simulink model "verificationGG"  (R2023b)
settings: Solver=ode5  StartTime=0.0  StopTime=5000  FixedStep=0.01  RelTol=1e-10  AbsTol=1e-11
values from neighbouring files (symbols this model uses):
  A_0 = A_B_LVLH*A_LVLH_ECI_0    [SAD_CALLER.m]    (also in veriAxilsym.m = eye(3))
  correct_g = [5.7   7.4   0      0     0 ... (first row only)    [SAD_CALLER.m]    (also in veriAxilsym.m)
  correct_h = [  0  -25.9     0       0      0 ... (first row only)    [SAD_CALLER.m]    (also in veriAxilsym.m)
  g_nm = [-29404.8 -1450.9     0      0     0 ... (first row only)    [SAD_CALLER.m]    (also in veriAxilsym.m)
  h_nm = [  0  4652.5      0      0       0 ... (first row only)    [SAD_CALLER.m]    (also in veriAxilsym.m)
  I = I_a+diag([0,4*M_a*x_cm^2,4*M_a*x_cm^2])+I_c+diag([0,M_c*d_cc_cm^2,M_c*d_cc_cm^2])+I_p+diag([0,6*M_p*(d_cc+d_cc_cm)^2,6*M_p*(d_cc-d_cc_cm)^2])    [SAD_CALLER.m]    (also in veriAxilsym.m = diag(I))
  Inv_I = inv(I)    [SAD_CALLER.m]    (also in veriAxilsym.m = pinv(I))
  J2 = 1.082626925638815e-3    (= 0.00108262692564)    [SAD_CALLER.m]    (also in veriAxilsym.m)
  m_sc_body = [1;1;1]*10e-3*M_tot/sqrt(3)    [SAD_CALLER.m]    (also in veriAxilsym.m)
  mu_E = 3.986004418e5    (= 398600.4418)    [SAD_CALLER.m]    (also in veriAxilsym.m = 398600)
  omega_E = 2*pi/(24*60*60)    (= 7.27220521664e-05)    [SAD_CALLER.m]    (also in veriAxilsym.m)
  omega_sc_0 = [0,0,n]    [SAD_CALLER.m]    (also in veriAxilsym.m = [0; 0; 0])
  R_E_eqtr = 6378.1363    [SAD_CALLER.m]    (also in veriAxilsym.m)
  rr_Esc_0 = s(end,(1:3))'    [SAD_CALLER.m]    (also in veriAxilsym.m = [7070.6; 0; 0])
  smith_norm = zeros(4,5)    [SAD_CALLER.m]    (also in veriAxilsym.m)
  theta_G0 = mod(theta_G_Winter_solstice+omega_E*t_elapsed,2*pi)    [SAD_CALLER.m]    (also in veriAxilsym.m)
  vv_Esc_0 = s(end,(4:6))'    [SAD_CALLER.m]    (also in veriAxilsym.m = [0; 7.4338; 0])
undefined symbols (not defined in the file or in its folder): omega_0
libraries: matrix_library x4, simulink_extras x1
settings Model: Creator=WinUser  LastModifiedBy=a1pab

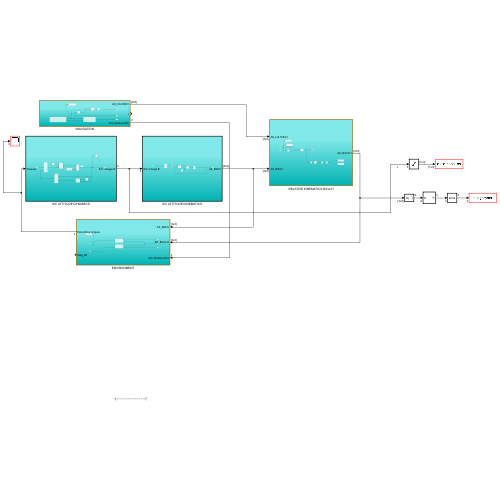
[thumbnail: Simulink's stored preview of the top-level diagram]
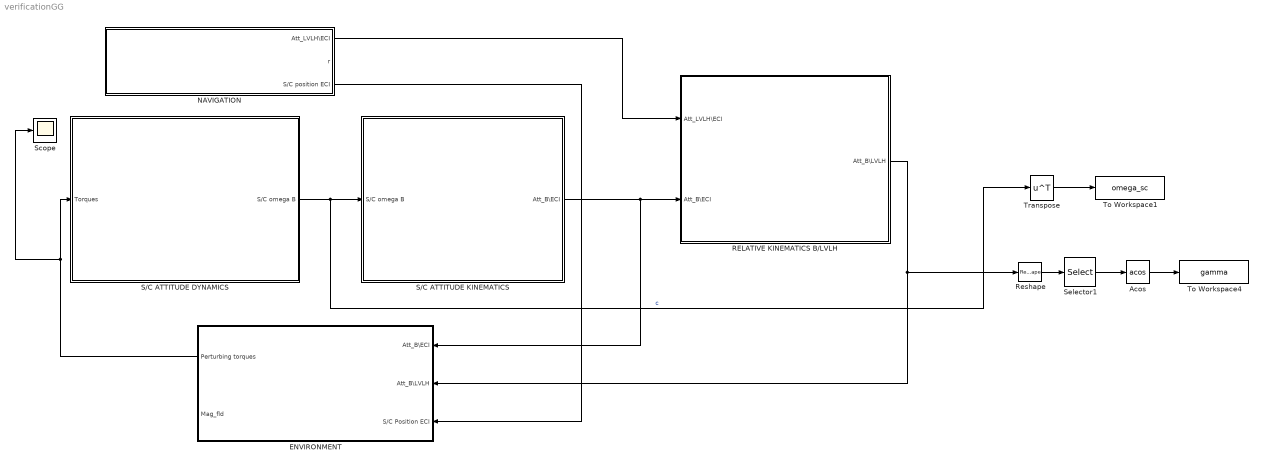
== system verificationGG ==
  Acos : Trigonometry  Operator=acos
  ENVIRONMENT : Subsystem
  NAVIGATION : Subsystem
  RELATIVE KINEMATICS B/LVLH : Subsystem
  Reshape : Reshape
  S/C ATTITUDE DYNAMICS : Subsystem
  S/C ATTITUDE KINEMATICS : Subsystem
  Scope : Scope
  Selector1 : Selector  InputPortWidth=9  IndexOptions=Index vector (dialog)  Indices=[1,5,9]  OutputSizes=1
  To Workspace1 : ToWorkspace  VariableName=omega_sc  SampleTime=-1
      settings: Save2DSignal=2-D array (concatenate along first dimension)
  To Workspace4 : ToWorkspace  VariableName=gamma  SampleTime=-1
      settings: Save2DSignal=2-D array (concatenate along first dimension)
  Transpose : Math  Operator=transpose
  wires:
  ? -> ?
  NAVIGATION/1(Att_LVLH\ECI) -> RELATIVE KINEMATICS B/LVLH/1(Att_LVLH\ECI)
  NAVIGATION/3(S/C position ECI) -> ENVIRONMENT/3(S/C Position ECI)
  RELATIVE KINEMATICS B/LVLH/1(Att_B\LVLH) -> Reshape/1, ENVIRONMENT/2(Att_B\LVLH)
  S/C ATTITUDE DYNAMICS/1(S/C omega B) -> Transpose/1, S/C ATTITUDE KINEMATICS/1(S/C omega B)  "c"
  Transpose/1 -> To Workspace1/1
  Selector1/1 -> Acos/1
  Reshape/1 -> Selector1/1
  Acos/1 -> To Workspace4/1
  S/C ATTITUDE KINEMATICS/1(Att_B\ECI) -> ENVIRONMENT/1(Att_B\ECI), RELATIVE KINEMATICS B/LVLH/2(Att_B\ECI)
  ENVIRONMENT/1(Perturbing torques) -> S/C ATTITUDE DYNAMICS/1(Torques), Scope/1

== system verificationGG/ENVIRONMENT ==
  Att_B\ECI : Inport
  Att_B\LVLH : Inport  Port=2
  S/C Position ECI : Inport  Port=3
  Gravity Gradient : Subsystem
  Magnetic Torque : Subsystem
  Sum : Sum  Inputs=+|+
  To Workspace1 : ToWorkspace  VariableName=ext_perturbations  SampleTime=-1
  Perturbing torques : Outport
  Mag_fld : Outport  Port=2
  wires:
  S/C Position ECI/1 -> Gravity Gradient/2(S/C Position), Magnetic Torque/1("[km]")
  Att_B\ECI/1 -> Magnetic Torque/2(True Attitude B\N)
  Att_B\LVLH/1 -> Gravity Gradient/1(Att_B\L)
  Gravity Gradient/1(GG_Torque) -> Sum/1
  Sum/1 -> To Workspace1/1, Perturbing torques/1
  Magnetic Torque/2(Mag_fld) -> Mag_fld/1

== system verificationGG/NAVIGATION ==
  LVLH Kinematics : Subsystem
  Matrix Multiply : Product  Multiplication=Matrix(*)
  S/C Orbit propagation : Subsystem
  Sqrt : Sqrt
  To Workspace4 : ToWorkspace  VariableName=position  SampleTime=-1
      settings: Save2DSignal=2-D array (concatenate along first dimension)
  Transpose : Math  Operator=transpose
  Att_LVLH\ECI : Outport
  r : Outport  Port=2
  S/C position ECI : Outport  Port=3
  wires:
  S/C Orbit propagation/2(S/C Velocity ECI) -> LVLH Kinematics/2(velocity)  "[km/s]"
  LVLH Kinematics/1(Att_LVLH\ECI) -> Att_LVLH\ECI/1
  Matrix Multiply/1 -> Sqrt/1
  Sqrt/1 -> r/1
  Transpose/1 -> Matrix Multiply/1
  S/C Orbit propagation/1(S/C Posiion ECI) -> To Workspace4/1, Matrix Multiply/2, Transpose/1, S/C position ECI/1, LVLH Kinematics/1(position)

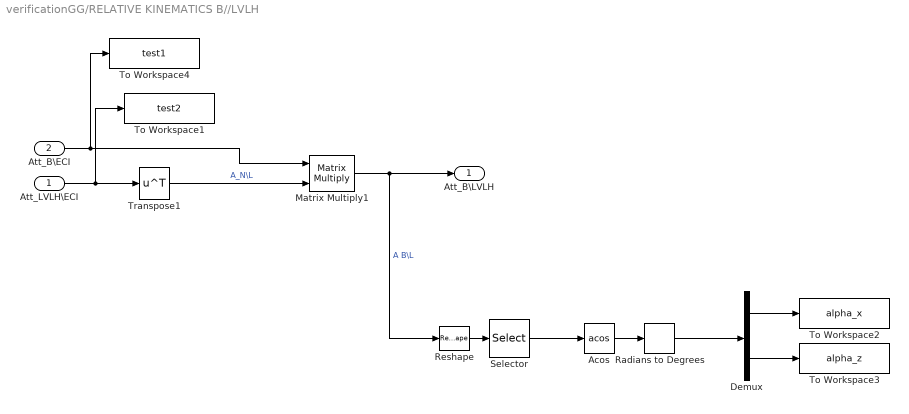
== system verificationGG/RELATIVE KINEMATICS B//LVLH ==
  Att_LVLH\ECI : Inport
  Att_B\ECI : Inport  Port=2
  Acos : Trigonometry  Operator=acos
  Demux : Demux  Outputs=2
  Matrix Multiply1 : Product  Multiplication=Matrix(*)
  Radians to Degrees : simulink_extras/Transformations/Radians to Degrees
  Reshape : Reshape
  Selector : Selector  InputPortWidth=9  IndexOptions=Index vector (dialog)  Indices=[1,9]  OutputSizes=1
  To Workspace1 : ToWorkspace  VariableName=test2  SampleTime=-1
      settings: Save2DSignal=2-D array (concatenate along first dimension)
  To Workspace2 : ToWorkspace  VariableName=alpha_x  SampleTime=-1
      settings: Save2DSignal=2-D array (concatenate along first dimension)
  To Workspace3 : ToWorkspace  VariableName=alpha_z  SampleTime=-1
      settings: Save2DSignal=2-D array (concatenate along first dimension)
  To Workspace4 : ToWorkspace  VariableName=test1  SampleTime=-1
      settings: Save2DSignal=2-D array (concatenate along first dimension)
  Transpose1 : Math  Operator=transpose
  Att_B\LVLH : Outport
  wires:
  Transpose1/1 -> Matrix Multiply1/2  "A_N\\L"
  Matrix Multiply1/1 -> Reshape/1, Att_B\LVLH/1  "A B\\L"
  Att_B\ECI/1 -> To Workspace4/1, Matrix Multiply1/1
  Att_LVLH\ECI/1 -> To Workspace1/1, Transpose1/1
  Demux/2 -> To Workspace3/1
  Demux/1 -> To Workspace2/1
  Selector/1 -> Acos/1
  Reshape/1 -> Selector/1
  Radians to Degrees/1 -> Demux/1
  Acos/1 -> Radians to Degrees/1

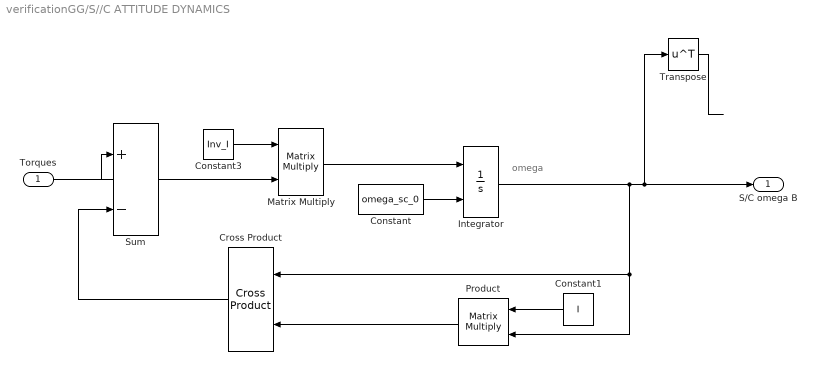
== system verificationGG/S//C ATTITUDE DYNAMICS ==
  note: omega
  Torques : Inport
  Constant : Constant  Value=omega_sc_0
  Constant1 : Constant  Value=I  VectorParams1D=off
  Constant3 : Constant  Value=Inv_I  VectorParams1D=off
  Cross Product : matrix_library/Cross Product
  Integrator : Integrator  InitialConditionSource=external  InitialCondition=omega_0
  Matrix Multiply : Product  Multiplication=Matrix(*)
  Product : Product  Multiplication=Matrix(*)
  Sum : Sum  Inputs=|+-
  Transpose : Math  Operator=transpose
  S/C omega B : Outport
  wires:
  Constant3/1 -> Matrix Multiply/1
  Constant/1 -> Integrator/2
  Sum/1 -> Matrix Multiply/2
  Cross Product/1 -> Sum/2
  Integrator/1 -> S/C omega B/1, Transpose/1, Cross Product/1, Product/2
  Constant1/1 -> Product/1
  Matrix Multiply/1 -> Integrator/1
  Torques/1 -> Sum/1
  Product/1 -> Cross Product/2
  Transpose/1 -> ?

== system verificationGG/S//C ATTITUDE KINEMATICS ==
  S/C omega B : Inport
  1st order orthon. : Subsystem
  Angular velocity tensor : Subsystem
  Constant3 : Constant  Value=A_0
  Gain : Gain  Gain=-1
  Integrator1 : Integrator  InitialConditionSource=external  InitialCondition=omega_0
  Matrix Multiply : Product  Multiplication=Matrix(*)
  Att_B\ECI : Outport
  wires:
  Constant3/1 -> Integrator1/2
  S/C omega B/1 -> Angular velocity tensor/1(In1)  "omega B\\N"
  1st order orthon./1(Out1) -> Att_B\ECI/1, Matrix Multiply/2  "True Attitude B\\N"
  Integrator1/1 -> 1st order orthon./1(In1)
  Matrix Multiply/1 -> Integrator1/1
  Gain/1 -> Matrix Multiply/1
  Angular velocity tensor/1(Out1) -> Gain/1

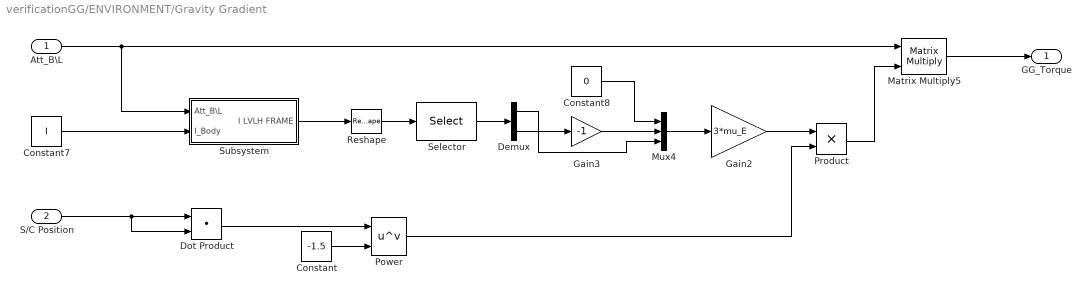
== system verificationGG/ENVIRONMENT/Gravity Gradient ==
  Att_B\L : Inport
  S/C Position : Inport  Port=2
  Constant : Constant  Value=-1.5
  Constant7 : Constant  Value=I
  Constant8 : Constant  Value=0
  Demux : Demux  Outputs=2
  Dot Product : DotProduct  OutDataTypeStr=Inherit: Inherit via internal rule
  Gain2 : Gain  Gain=3*mu_E
  Gain3 : Gain  Gain=-1
  Matrix Multiply5 : Product  Multiplication=Matrix(*)
  Mux4 : Mux  Inputs=3
  Power : Math  Operator=pow
  Product : Product
  Reshape : Reshape
  Selector : Selector  InputPortWidth=9  IndexOptions=Index vector (dialog)  Indices=[2,3]  OutputSizes=1
  Subsystem : Subsystem
  GG_Torque : Outport
  wires:
  Selector/1 -> Demux/1
  Reshape/1 -> Selector/1
  Att_B\L/1 -> Subsystem/1(Att_B\L), Matrix Multiply5/1
  Mux4/1 -> Gain2/1
  Constant8/1 -> Mux4/1
  Demux/1 -> Mux4/3
  Matrix Multiply5/1 -> GG_Torque/1
  Demux/2 -> Gain3/1
  Gain3/1 -> Mux4/2
  Constant7/1 -> Subsystem/2(I_Body)
  Subsystem/1(I LVLH FRAME) -> Reshape/1
  Gain2/1 -> Product/1
  Product/1 -> Matrix Multiply5/2
  S/C Position/1 -> Dot Product/1, Dot Product/2
  Dot Product/1 -> Power/1
  Constant/1 -> Power/2
  Power/1 -> Product/2

== system verificationGG/ENVIRONMENT/Magnetic Torque ==
  "[km]" : Inport
  True Attitude B\N : Inport  Port=2
  Cartesian 2 spherical : Subsystem
  Constant1 : Constant  Value=m_sc_body
  MAGNETIC TORQUE in BODY : Subsystem
  MF_Torque : Outport
  Mag_fld : Outport  Port=2
  wires:
  "[km]"/1 -> Cartesian 2 spherical/1("[km]")
  Cartesian 2 spherical/1(LST) -> MAGNETIC TORQUE in BODY/1(local siderial time)
  Cartesian 2 spherical/2(Long) -> MAGNETIC TORQUE in BODY/2(longitude)  "[rad]"
  Cartesian 2 spherical/3(radius) -> MAGNETIC TORQUE in BODY/3(r)
  Constant1/1 -> MAGNETIC TORQUE in BODY/6(a)
  MAGNETIC TORQUE in BODY/1(M) -> MF_Torque/1
  Cartesian 2 spherical/4(lat) -> MAGNETIC TORQUE in BODY/4(latitude)  "[rad]"
  True Attitude B\N/1 -> MAGNETIC TORQUE in BODY/5(True_Att_B\N)
  MAGNETIC TORQUE in BODY/2(Mag_fld) -> Mag_fld/1

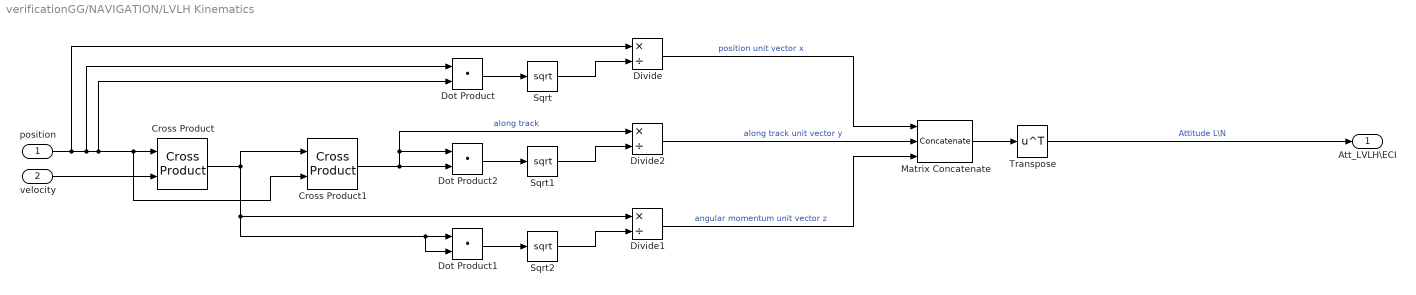
== system verificationGG/NAVIGATION/LVLH Kinematics ==
  position : Inport
  velocity : Inport  Port=2
  Cross Product : matrix_library/Cross Product
  Cross Product1 : matrix_library/Cross Product
  Divide : Product  Inputs=*/
  Divide1 : Product  Inputs=*/
  Divide2 : Product  Inputs=*/
  Dot Product : DotProduct  OutDataTypeStr=Inherit: Inherit via internal rule
  Dot Product1 : DotProduct  OutDataTypeStr=Inherit: Inherit via internal rule
  Dot Product2 : DotProduct  OutDataTypeStr=Inherit: Inherit via internal rule
  Matrix Concatenate : Concatenate  NumInputs=3  Mode=Multidimensional array  ConcatenateDimension=2
  Sqrt : Sqrt
  Sqrt1 : Sqrt
  Sqrt2 : Sqrt
  Transpose : Math  Operator=transpose
  Att_LVLH\ECI : Outport
  wires:
  Divide2/1 -> Matrix Concatenate/2  "along track unit vector y"
  Sqrt/1 -> Divide/2
  Cross Product/1 -> Dot Product1/2, Dot Product1/1, Divide1/1, Cross Product1/1
  Cross Product1/1 -> Divide2/1, Dot Product2/1, Dot Product2/2  "along track"
  Divide/1 -> Matrix Concatenate/1  "position unit vector x"
  position/1 -> Divide/1, Dot Product/1, Dot Product/2, Cross Product1/2, Cross Product/1
  velocity/1 -> Cross Product/2
  Sqrt2/1 -> Divide1/2
  Matrix Concatenate/1 -> Transpose/1
  Sqrt1/1 -> Divide2/2
  Divide1/1 -> Matrix Concatenate/3  "angular momentum unit vector z"
  Dot Product1/1 -> Sqrt2/1
  Dot Product/1 -> Sqrt/1
  Dot Product2/1 -> Sqrt1/1
  Transpose/1 -> Att_LVLH\ECI/1  "Attitude L\\N"

== system verificationGG/NAVIGATION/S//C Orbit propagation ==
  Constant5 : Constant  Value=vv_Esc_0
  Constant6 : Constant  Value=rr_Esc_0
  Integrator2 : Integrator  InitialConditionSource=external
  Integrator3 : Integrator  InitialConditionSource=external
  J2 perturbation : Subsystem
  Keplerian motion : Subsystem
  Sum : Sum  Inputs=|+-
  To Workspace : ToWorkspace  VariableName=RR_Esc  SampleTime=-1
  To Workspace1 : ToWorkspace  VariableName=VV_Esc  SampleTime=-1
  S/C Posiion ECI : Outport
  S/C Velocity ECI : Outport  Port=2
  wires:
  J2 perturbation/1(J2 acceleration) -> Sum/1
  Keplerian motion/1(Keplerian acceleration) -> Sum/2
  Constant5/1 -> Integrator2/2
  Integrator2/1 -> To Workspace1/1, S/C Velocity ECI/1, Integrator3/1  "dr"
  Constant6/1 -> Integrator3/2
  Sum/1 -> Integrator2/1  "ddr"
  Integrator3/1 -> S/C Posiion ECI/1, J2 perturbation/1(Position vector), Keplerian motion/1(Position vector), To Workspace/1  "r"

== system verificationGG/S//C ATTITUDE KINEMATICS/1st order orthon. ==
  In1 : Inport
  Gain1 : Gain  Gain=3/2
  Gain2 : Gain  Gain=1/2
  Matrix Multiply1 : Product  Multiplication=Matrix(*)
  Matrix Multiply2 : Product  Multiplication=Matrix(*)
  Sum1 : Sum  Inputs=|+-
  Transpose : Math  Operator=transpose
  Out1 : Outport
  wires:
  Gain1/1 -> Sum1/1
  In1/1 -> Matrix Multiply2/2, Transpose/1, Gain2/1, Gain1/1
  Transpose/1 -> Matrix Multiply1/2
  Matrix Multiply2/1 -> Sum1/2
  Matrix Multiply1/1 -> Matrix Multiply2/1
  Sum1/1 -> Out1/1
  Gain2/1 -> Matrix Multiply1/1

== system verificationGG/S//C ATTITUDE KINEMATICS/Angular velocity tensor ==
  In1 : Inport
  Constant : Constant  Value=0
  Demux1 : Demux  Outputs=3
  Gain3 : Gain  Gain=-1
  Gain4 : Gain  Gain=-1
  Gain5 : Gain  Gain=-1
  Mux3 : Mux  Inputs=3
  Mux4 : Mux  Inputs=3
  Mux5 : Mux  Inputs=3
  Vector Concatenate : Concatenate  NumInputs=3  Mode=Multidimensional array  ConcatenateDimension=2
  Out1 : Outport
  wires:
  In1/1 -> Demux1/1
  Constant/1 -> Mux3/1, Mux4/2, Mux5/3
  Demux1/3 -> Gain4/1, Mux3/2
  Demux1/2 -> Gain3/1, Mux5/1
  Gain3/1 -> Mux3/3
  Gain4/1 -> Mux4/1
  Mux4/1 -> Vector Concatenate/2
  Demux1/1 -> Gain5/1, Mux4/3
  Gain5/1 -> Mux5/2
  Mux5/1 -> Vector Concatenate/3
  Mux3/1 -> Vector Concatenate/1
  Vector Concatenate/1 -> Out1/1

== system verificationGG/ENVIRONMENT/Gravity Gradient/Subsystem ==
  Att_B\L : Inport
  I_Body : Inport  Port=2
  Matrix Multiply3 : Product  Multiplication=Matrix(*)
  Matrix Multiply4 : Product  Multiplication=Matrix(*)
  Transpose2 : Math  Operator=transpose
  I LVLH FRAME : Outport
  wires:
  Matrix Multiply3/1 -> I LVLH FRAME/1  "I LVLH FRAME"
  Matrix Multiply4/1 -> Matrix Multiply3/1
  I_Body/1 -> Matrix Multiply4/2
  Att_B\L/1 -> Transpose2/1, Matrix Multiply3/2
  Transpose2/1 -> Matrix Multiply4/1

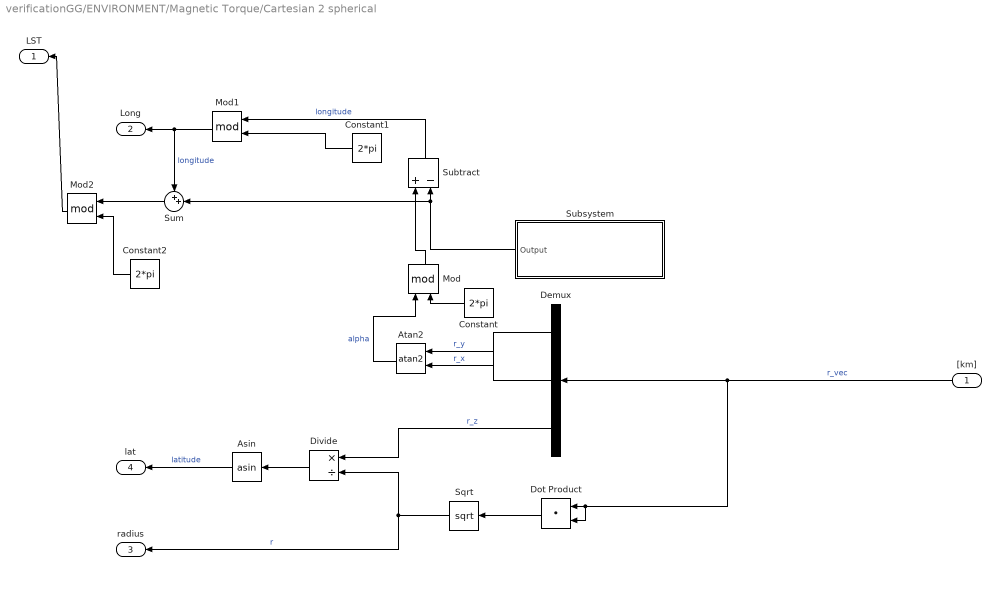
== system verificationGG/ENVIRONMENT/Magnetic Torque/Cartesian 2 spherical ==
  "[km]" : Inport
  Asin : Trigonometry  Operator=asin
  Atan2 : Trigonometry  Operator=atan2
  Constant : Constant  Value=2*pi
  Constant1 : Constant  Value=2*pi
  Constant2 : Constant  Value=2*pi
  Demux : Demux  Outputs=3
  Divide : Product  Inputs=*/
  Dot Product : DotProduct  OutDataTypeStr=Inherit: Inherit via internal rule
  Mod : Math  Operator=mod
  Mod1 : Math  Operator=mod
  Mod2 : Math  Operator=mod
  Sqrt : Sqrt
  Subsystem : Subsystem
  Subtract : Sum  Inputs=+-
  Sum : Sum  Inputs=++|
  LST : Outport
  Long : Outport  Port=2
  radius : Outport  Port=3
  lat : Outport  Port=4
  wires:
  "[km]"/1 -> Dot Product/2, Dot Product/1, Demux/1  "r_vec"
  Demux/2 -> Atan2/1  "r_y"
  Demux/1 -> Atan2/2  "r_x"
  Subsystem/1(Output) -> Sum/2, Subtract/2
  Dot Product/1 -> Sqrt/1
  Demux/3 -> Divide/1  "r_z"
  Sqrt/1 -> radius/1, Divide/2  "r"
  Divide/1 -> Asin/1
  Asin/1 -> lat/1  "latitude"
  Constant1/1 -> Mod1/2
  Subtract/1 -> Mod1/1  "longitude"
  Mod/1 -> Subtract/1
  Atan2/1 -> Mod/1  "alpha"
  Constant/1 -> Mod/2
  Mod1/1 -> Long/1, Sum/1  "longitude"
  Sum/1 -> Mod2/1
  Constant2/1 -> Mod2/2
  Mod2/1 -> LST/1

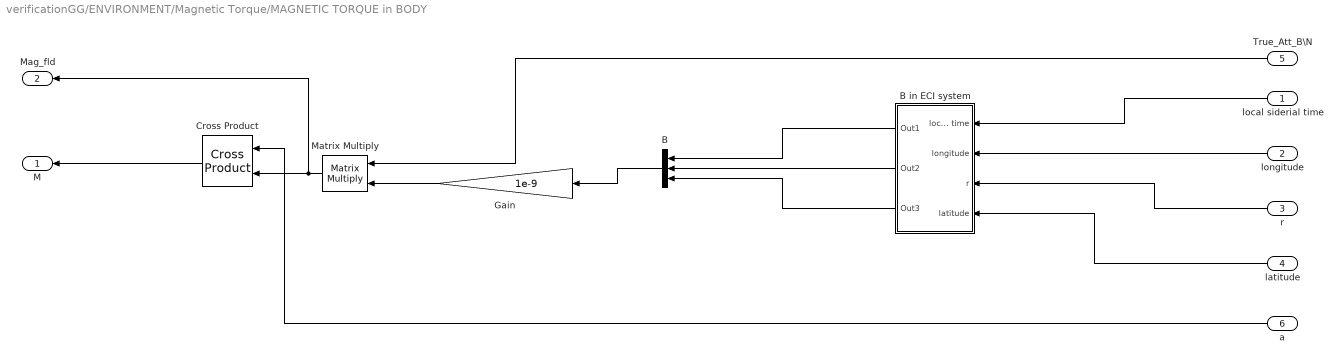
== system verificationGG/ENVIRONMENT/Magnetic Torque/MAGNETIC TORQUE in BODY ==
  local siderial time : Inport
  longitude : Inport  Port=2
  r : Inport  Port=3
  latitude : Inport  Port=4
  True_Att_B\N : Inport  Port=5
  a : Inport  Port=6
  B : Concatenate  NumInputs=3
  B in ECI system : Subsystem
  Cross Product : matrix_library/Cross Product
  Gain : Gain  Gain=1e-9
  Matrix Multiply : Product  Multiplication=Matrix(*)
  M : Outport
  Mag_fld : Outport  Port=2
  wires:
  B in ECI system/1(Out1) -> B/1
  a/1 -> Cross Product/1
  B in ECI system/2(Out2) -> B/2
  r/1 -> B in ECI system/3(r)
  local siderial time/1 -> B in ECI system/1(local siderial time)
  latitude/1 -> B in ECI system/4(latitude)
  B in ECI system/3(Out3) -> B/3
  Cross Product/1 -> M/1
  longitude/1 -> B in ECI system/2(longitude)
  B/1 -> Gain/1
  True_Att_B\N/1 -> Matrix Multiply/1
  Gain/1 -> Matrix Multiply/2
  Matrix Multiply/1 -> Mag_fld/1, Cross Product/2

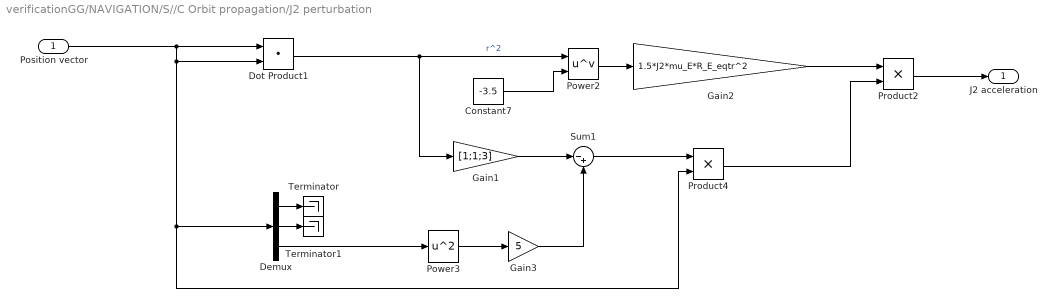
== system verificationGG/NAVIGATION/S//C Orbit propagation/J2 perturbation ==
  Position vector : Inport
  Constant7 : Constant  Value=-3.5
  Demux : Demux  Outputs=3
  Dot Product1 : DotProduct  OutDataTypeStr=Inherit: Inherit via internal rule
  Gain1 : Gain  Gain=[1;1;3]
  Gain2 : Gain  Gain=1.5*J2*mu_E*R_E_eqtr^2
  Gain3 : Gain  Gain=5
  Power2 : Math  Operator=pow
  Power3 : Math  Operator=square
  Product2 : Product
  Product4 : Product
  Sum1 : Sum  Inputs=|-+
  Terminator : Terminator
  Terminator1 : Terminator
  J2 acceleration : Outport
  wires:
  Gain3/1 -> Sum1/2
  Power2/1 -> Gain2/1
  Dot Product1/1 -> Power2/1, Gain1/1  "r^2"
  Demux/1 -> Terminator/1
  Gain1/1 -> Sum1/1
  Gain2/1 -> Product2/1
  Demux/3 -> Power3/1
  Power3/1 -> Gain3/1
  Product4/1 -> Product2/2
  Demux/2 -> Terminator1/1
  Constant7/1 -> Power2/2
  Product2/1 -> J2 acceleration/1
  Position vector/1 -> Demux/1, Product4/2, Dot Product1/2, Dot Product1/1
  Sum1/1 -> Product4/1

== system verificationGG/NAVIGATION/S//C Orbit propagation/Keplerian motion ==
  Position vector : Inport
  Constant : Constant  Value=-1.5
  Dot Product2 : DotProduct  OutDataTypeStr=Inherit: Inherit via internal rule
  Gain1 : Gain  Gain=mu_E
  Power : Math  Operator=pow
  Product1 : Product
  Keplerian acceleration : Outport
  wires:
  Position vector/1 -> Product1/2, Dot Product2/2, Dot Product2/1
  Power/1 -> Gain1/1
  Gain1/1 -> Product1/1
  Product1/1 -> Keplerian acceleration/1
  Constant/1 -> Power/2
  Dot Product2/1 -> Power/1  "r^2"

== system verificationGG/ENVIRONMENT/Magnetic Torque/Cartesian 2 spherical/Subsystem ==
  Clock : Clock
  Constant : Constant  Value=theta_G0
  Constant1 : Constant  Value=omega_E
  Constant2 : Constant  Value=2*pi
  Mod : Math  Operator=mod
  Product : Product
  Sum : Sum  Inputs=|++
  Output : Outport
  wires:
  Constant/1 -> Sum/1
  Product/1 -> Sum/2
  Clock/1 -> Product/2
  Sum/1 -> Mod/1  "theta_G(t)"
  Constant1/1 -> Product/1
  Constant2/1 -> Mod/2
  Mod/1 -> Output/1

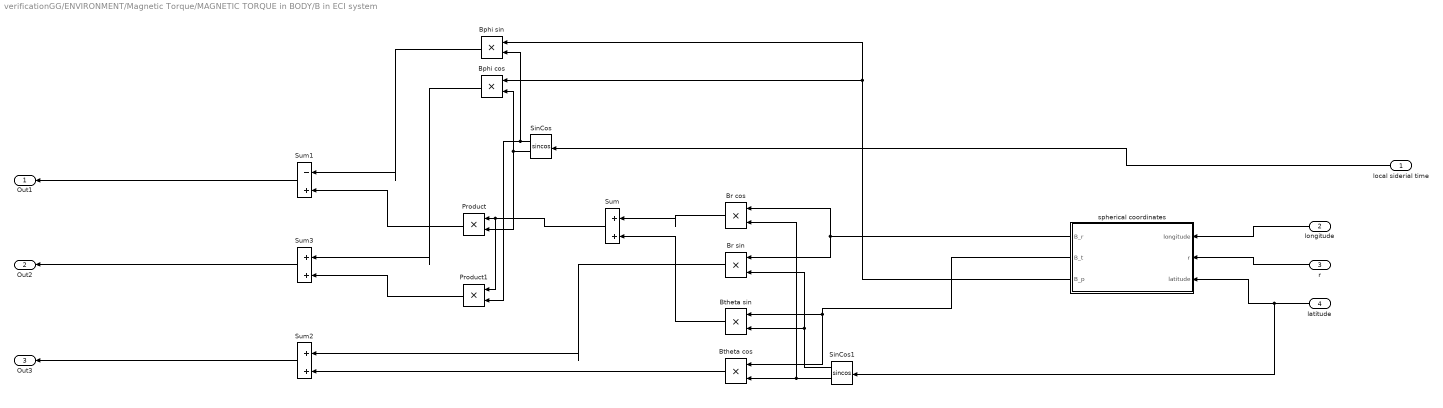
== system verificationGG/ENVIRONMENT/Magnetic Torque/MAGNETIC TORQUE in BODY/B in ECI system ==
  local siderial time : Inport
  longitude : Inport  Port=2
  r : Inport  Port=3
  latitude : Inport  Port=4
  Bphi cos : Product
  Bphi sin : Product
  Br cos : Product
  Br sin : Product
  Btheta cos : Product
  Btheta sin : Product
  Product : Product
  Product1 : Product
  SinCos : Trigonometry  Operator=sincos
  SinCos1 : Trigonometry  Operator=sincos
  Sum : Sum  Inputs=|++
  Sum1 : Sum  Inputs=|-+
  Sum2 : Sum  Inputs=|++
  Sum3 : Sum  Inputs=|++
  spherical coordinates : Subsystem
  Out1 : Outport
  Out2 : Outport  Port=2
  Out3 : Outport  Port=3
  wires:
  Sum3/1 -> Out2/1
  Sum1/1 -> Out1/1
  Bphi sin/1 -> Sum1/1
  Btheta sin/1 -> Sum/2
  Sum2/1 -> Out3/1
  Product1/1 -> Sum3/2
  SinCos1/2 -> Btheta cos/2, Br cos/2
  r/1 -> spherical coordinates/2(r)
  latitude/1 -> SinCos1/1, spherical coordinates/3(latitude)
  spherical coordinates/1(B_r) -> Br cos/1, Br sin/1
  Br sin/1 -> Sum2/1
  longitude/1 -> spherical coordinates/1(longitude)
  local siderial time/1 -> SinCos/1
  spherical coordinates/2(B_t) -> Btheta sin/1, Btheta cos/1
  Sum/1 -> Product1/1, Product/1
  Br cos/1 -> Sum/1
  Btheta cos/1 -> Sum2/2
  SinCos1/1 -> Btheta sin/2, Br sin/2
  SinCos/2 -> Bphi cos/2, Product/2
  Bphi cos/1 -> Sum3/1
  SinCos/1 -> Bphi sin/2, Product1/2
  Product/1 -> Sum1/2
  spherical coordinates/3(B_p) -> Bphi sin/1, Bphi cos/1

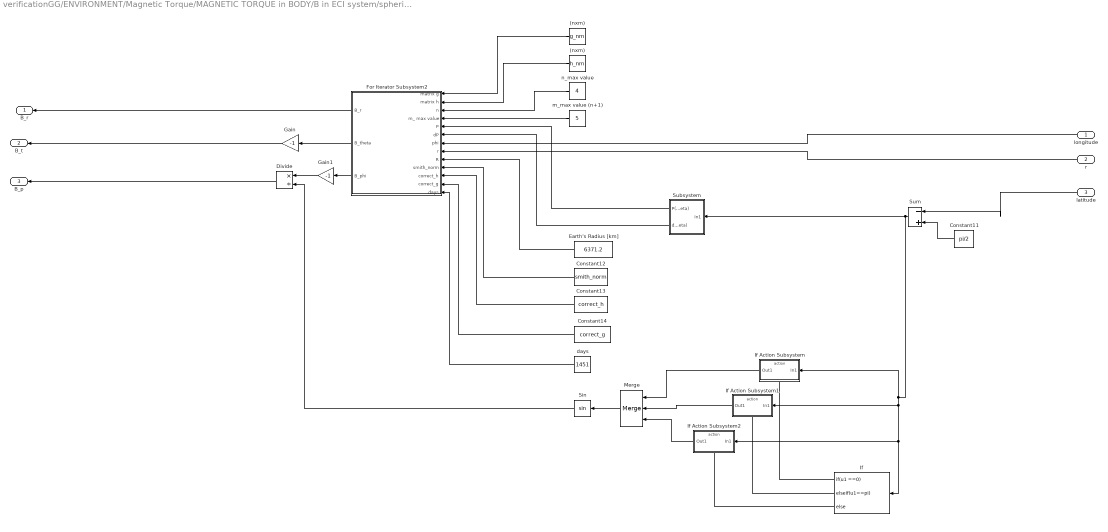
== system verificationGG/ENVIRONMENT/Magnetic Torque/MAGNETIC TORQUE in BODY/B in ECI system/spherical coordinates ==
  longitude : Inport
  r : Inport  Port=2
  latitude : Inport  Port=3
  " (nxm)" : Constant  Value=g_nm
  (nxm) : Constant  Value=h_nm
  Constant11 : Constant  Value=pi/2
  Constant12 : Constant  Value=smith_norm
  Constant13 : Constant  Value=correct_h
  Constant14 : Constant  Value=correct_g
  Divide : Product  Inputs=*/
  Earth's Radius [km] : Constant  Value=6371.2
  For Iterator Subsystem2 : Subsystem  TreatAsAtomicUnit=on
  Gain : Gain  Gain=-1
  Gain1 : Gain  Gain=-1
  If : If  IfExpression=u1 ==0  ElseIfExpressions=u1==pi
  If Action Subsystem : Subsystem  TreatAsAtomicUnit=on
  If Action Subsystem1 : Subsystem  TreatAsAtomicUnit=on
  If Action Subsystem2 : Subsystem  TreatAsAtomicUnit=on
  Merge : Merge  Inputs=3
  Sin : Trigonometry
  Subsystem : Subsystem
  Sum : Sum  Inputs=|-+
  days : Constant  Value=1451
  m_max value (n+1) : Constant  Value=5
  n_max value : Constant  Value=4  OutDataTypeStr=int32
  B_r : Outport
  B_t : Outport  Port=2
  B_p : Outport  Port=3
  wires:
  Divide/1 -> B_p/1
  Constant11/1 -> Sum/2
  Gain/1 -> B_t/1
  Subsystem/1(P(theta)) -> For Iterator Subsystem2/5(P)
  days/1 -> For Iterator Subsystem2/13(days)
  For Iterator Subsystem2/1(B_r) -> B_r/1
  n_max value/1 -> For Iterator Subsystem2/3(n)
  For Iterator Subsystem2/2(B_theta) -> Gain/1
  Constant13/1 -> For Iterator Subsystem2/11("correct_h ")
  Constant14/1 -> For Iterator Subsystem2/12(correct_g)
  r/1 -> For Iterator Subsystem2/8(r)
  longitude/1 -> For Iterator Subsystem2/7(phi)
  Subsystem/2(dP(theta)) -> For Iterator Subsystem2/6(dP)
  latitude/1 -> Sum/1
  Sin/1 -> Divide/2
  Constant12/1 -> For Iterator Subsystem2/10(smith_norm)
  Earth's Radius [km]/1 -> For Iterator Subsystem2/9(R)
  Gain1/1 -> Divide/1
  For Iterator Subsystem2/3(B_phi) -> Gain1/1
  m_max value (n+1)/1 -> For Iterator Subsystem2/4(m_ max value)
  " (nxm)"/1 -> For Iterator Subsystem2/1(matrix g)
  (nxm)/1 -> For Iterator Subsystem2/2(matrix h)
  If Action Subsystem1/1(Out1) -> Merge/2
  If Action Subsystem2/1(Out1) -> Merge/3
  If Action Subsystem/1(Out1) -> Merge/1
  Sum/1 -> If Action Subsystem/1(In1), If Action Subsystem2/1(In1), If/1, If Action Subsystem1/1(In1), Subsystem/1(In1)
  Merge/1 -> Sin/1
  If/3 -> If Action Subsystem2/Action
  If/1 -> If Action Subsystem/Action
  If/2 -> If Action Subsystem1/Action

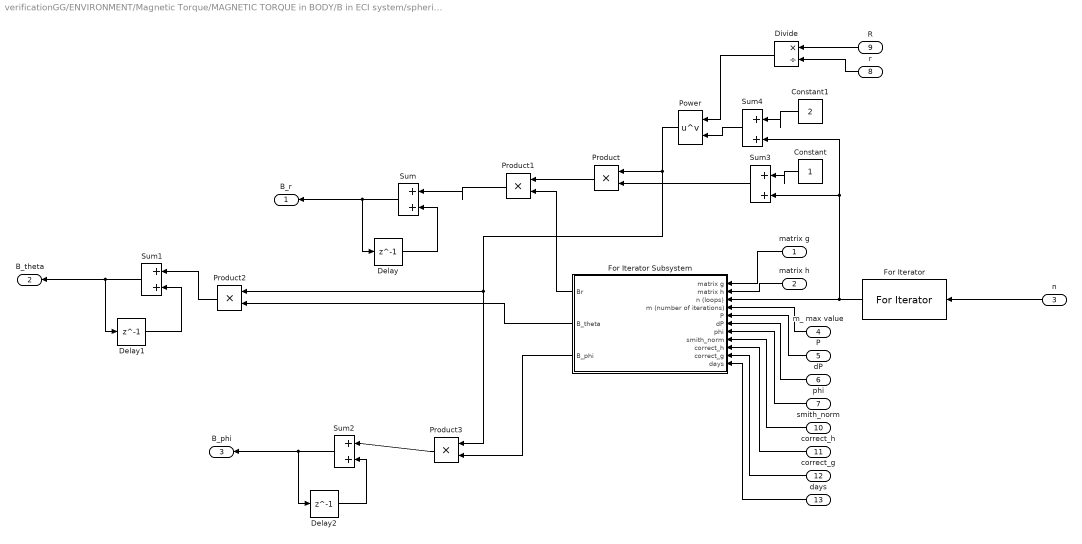
== system verificationGG/ENVIRONMENT/Magnetic Torque/MAGNETIC TORQUE in BODY/B in ECI system/spherical coordinates/For Iterator Subsystem2 ==
  matrix g : Inport
  matrix h : Inport  Port=2
  n : Inport  Port=3
  m_ max value : Inport  Port=4
  P : Inport  Port=5
  dP : Inport  Port=6
  phi : Inport  Port=7
  r : Inport  Port=8
  R : Inport  Port=9
  smith_norm : Inport  Port=10
  "correct_h " : Inport  Port=11
  correct_g : Inport  Port=12
  days : Inport  Port=13
  Constant : Constant
  Constant1 : Constant  Value=2
  Delay : Delay  DelayLength=1  InitialCondition=0
  Delay1 : Delay  DelayLength=1  InitialCondition=0
  Delay2 : Delay  DelayLength=1  InitialCondition=0
  Divide : Product  Inputs=*/
  For Iterator : ForIterator  ResetStates=reset  IterationSource=external
  For Iterator Subsystem : Subsystem  TreatAsAtomicUnit=on
  Power : Math  Operator=pow  OutputSignalType=real
  Product{,1..3} (4 alike) : Product
  Sum : Sum  Inputs=|++
  Sum1 : Sum  Inputs=|++
  Sum2 : Sum  Inputs=|++
  Sum3 : Sum  Inputs=|++  OutDataTypeStr=double
  Sum4 : Sum  Inputs=|++  OutDataTypeStr=double
  B_r : Outport
  B_theta : Outport  Port=2
  B_phi : Outport  Port=3
  wires:
  n/1 -> For Iterator/1
  Sum/1 -> Delay/1, B_r/1
  Delay/1 -> Sum/2
  matrix h/1 -> For Iterator Subsystem/2(matrix h)
  matrix g/1 -> For Iterator Subsystem/1(matrix g)
  For Iterator/1 -> Sum4/2, Sum3/2, For Iterator Subsystem/3(n (loops))
  m_ max value/1 -> For Iterator Subsystem/4(m (number of iterations))
  P/1 -> For Iterator Subsystem/5(P)
  dP/1 -> For Iterator Subsystem/6(dP)
  Sum1/1 -> Delay1/1, B_theta/1
  Delay1/1 -> Sum1/2
  Sum2/1 -> Delay2/1, B_phi/1
  Delay2/1 -> Sum2/2
  phi/1 -> For Iterator Subsystem/7(phi)
  Constant/1 -> Sum3/1
  R/1 -> Divide/1
  r/1 -> Divide/2
  Sum3/1 -> Product/2
  Divide/1 -> Power/1
  Power/1 -> Product/1, Product3/1, Product2/1
  Product/1 -> Product1/1
  For Iterator Subsystem/1(Br) -> Product1/2
  Product1/1 -> Sum/1
  Constant1/1 -> Sum4/1
  Sum4/1 -> Power/2
  smith_norm/1 -> For Iterator Subsystem/8(smith_norm)
  "correct_h "/1 -> For Iterator Subsystem/9("correct_h ")
  correct_g/1 -> For Iterator Subsystem/10(correct_g)
  days/1 -> For Iterator Subsystem/11(days)
  Product2/1 -> Sum1/1
  For Iterator Subsystem/2(B_theta) -> Product2/2
  Product3/1 -> Sum2/1
  For Iterator Subsystem/3(B_phi) -> Product3/2

== system verificationGG/ENVIRONMENT/Magnetic Torque/MAGNETIC TORQUE in BODY/B in ECI system/spherical coordinates/If Action Subsystem ==
  In1 : Inport
  Action Port : ActionPort  ActionPortLabel=if(u1 ==0)
  Constant : Constant  Value=0.0000001
  Sum : Sum  Inputs=|++
  Out1 : Outport
  wires:
  In1/1 -> Sum/1
  Sum/1 -> Out1/1
  Constant/1 -> Sum/2

== system verificationGG/ENVIRONMENT/Magnetic Torque/MAGNETIC TORQUE in BODY/B in ECI system/spherical coordinates/If Action Subsystem1 ==
  In1 : Inport
  Action Port : ActionPort  ActionPortLabel=elseif(u1==pi)
  Constant : Constant  Value=0.0000001
  Sum : Sum  Inputs=|++
  Out1 : Outport
  wires:
  In1/1 -> Sum/1
  Sum/1 -> Out1/1
  Constant/1 -> Sum/2

== system verificationGG/ENVIRONMENT/Magnetic Torque/MAGNETIC TORQUE in BODY/B in ECI system/spherical coordinates/If Action Subsystem2 ==
  In1 : Inport
  Action Port : ActionPort  ActionPortLabel=else
  Out1 : Outport
  wires:
  In1/1 -> Out1/1

== system verificationGG/ENVIRONMENT/Magnetic Torque/MAGNETIC TORQUE in BODY/B in ECI system/spherical coordinates/Subsystem ==
  In1 : Inport
  If : If  IfExpression=u1 ==0  ElseIfExpressions=u1==pi
  If Action Subsystem : Subsystem  TreatAsAtomicUnit=on
  If Action Subsystem1 : Subsystem  TreatAsAtomicUnit=on
  If Action Subsystem2 : Subsystem  TreatAsAtomicUnit=on
  Merge : Merge  Inputs=3
  P(v) : MATLAB Function  TreatAsAtomicUnit=on
  dP(v) : MATLAB Function  TreatAsAtomicUnit=on
  P(theta) : Outport
  dP(theta) : Outport  Port=2
  wires:
  dP(v)/1(y) -> dP(theta)/1
  If/2 -> If Action Subsystem1/Action
  P(v)/1(y) -> P(theta)/1
  If/1 -> If Action Subsystem/Action
  If Action Subsystem1/1(Out1) -> Merge/2
  If Action Subsystem/1(Out1) -> Merge/1
  Merge/1 -> dP(v)/1(u), P(v)/1(u)
  If Action Subsystem2/1(Out1) -> Merge/3
  In1/1 -> If Action Subsystem/1(In1), If Action Subsystem2/1(In1), If/1, If Action Subsystem1/1(In1)
  If/3 -> If Action Subsystem2/Action

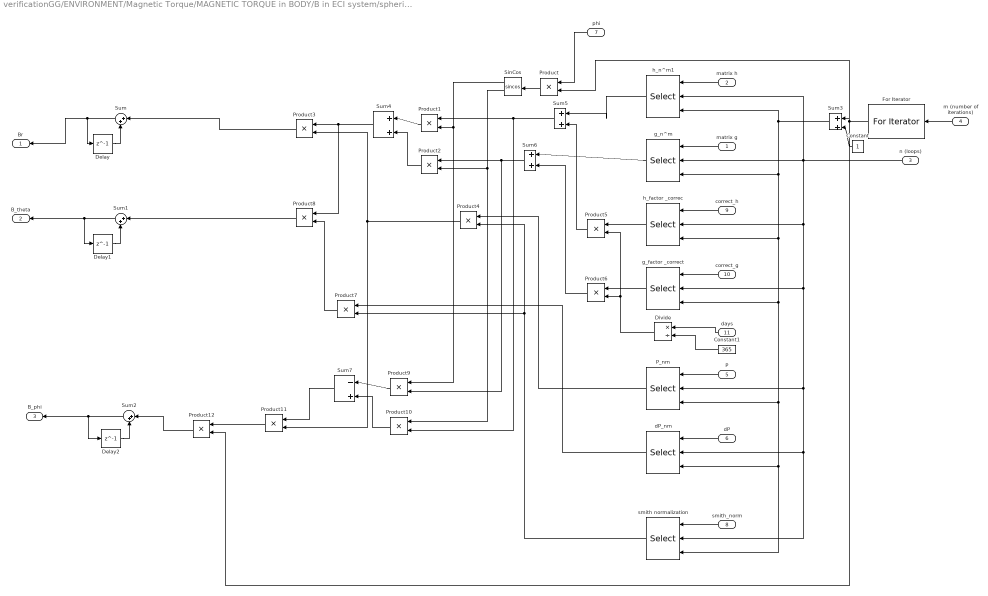
== system verificationGG/ENVIRONMENT/Magnetic Torque/MAGNETIC TORQUE in BODY/B in ECI system/spherical coordinates/For Iterator Subsystem2/For Iterator Subsystem ==
  matrix g : Inport
  matrix h : Inport  Port=2
  n (loops) : Inport  Port=3
  m (number of iterations) : Inport  Port=4
  P : Inport  Port=5
  dP : Inport  Port=6
  phi : Inport  Port=7
  smith_norm : Inport  Port=8
  "correct_h " : Inport  Port=9
  correct_g : Inport  Port=10
  days : Inport  Port=11
  Constant : Constant
  Constant1 : Constant  Value=365
  Delay : Delay  DelayLength=1  InitialCondition=0
  Delay1 : Delay  DelayLength=1  InitialCondition=0
  Delay2 : Delay  DelayLength=1  InitialCondition=0
  Divide : Product  Inputs=*/
  For Iterator : ForIterator  ResetStates=reset  IterationSource=external  IndexMode=Zero-based
  P_nm : Selector  NumberOfDimensions=2  InputPortWidth=6  IndexOptions=Starting index (port),Starting index (port)  Indices=[1 3],1  OutputSizes=1,1
  Product{,1..12} (13 alike) : Product
  SinCos : Trigonometry  Operator=sincos
  Sum{,1..6} (7 alike) : Sum  Inputs=|++
  Sum7 : Sum  Inputs=|-+
  dP_nm : Selector  NumberOfDimensions=2  InputPortWidth=6  IndexOptions=Starting index (port),Starting index (port)  Indices=[1 3],1  OutputSizes=1,1
  g_factor _correct : Selector  NumberOfDimensions=2  InputPortWidth=6  IndexOptions=Starting index (port),Starting index (port)  Indices=[1 3],1  OutputSizes=1,1
  g_n^m : Selector  NumberOfDimensions=2  InputPortWidth=6  IndexOptions=Starting index (port),Starting index (port)  Indices=[1 3],1  OutputSizes=1,1
  h_factor _correc : Selector  NumberOfDimensions=2  InputPortWidth=6  IndexOptions=Starting index (port),Starting index (port)  Indices=[1 3],1  OutputSizes=1,1
  h_n^m1 : Selector  NumberOfDimensions=2  InputPortWidth=6  IndexOptions=Starting index (port),Starting index (port)  Indices=[1 3],1  OutputSizes=1,1
  smith normalization : Selector  NumberOfDimensions=2  InputPortWidth=6  IndexOptions=Starting index (port),Starting index (port)  Indices=[1 3],1  OutputSizes=1,1
  Br : Outport
  B_theta : Outport  Port=2
  B_phi : Outport  Port=3
  wires:
  Sum/1 -> Br/1, Delay/1
  Delay/1 -> Sum/2
  m (number of iterations)/1 -> For Iterator/1
  matrix g/1 -> g_n^m/1
  matrix h/1 -> h_n^m1/1
  P/1 -> P_nm/1
  dP/1 -> dP_nm/1
  Sum1/1 -> B_theta/1, Delay1/1
  Delay1/1 -> Sum1/2
  Sum2/1 -> B_phi/1, Delay2/1
  Delay2/1 -> Sum2/2
  For Iterator/1 -> Product/2, Product12/2, Sum3/1
  Constant/1 -> Sum3/2
  phi/1 -> Product/1
  Product/1 -> SinCos/1
  Product1/1 -> Sum4/1
  Product2/1 -> Sum4/2
  Sum4/1 -> Product8/1, Product3/1
  P_nm/1 -> Product4/1
  Product3/1 -> Sum/1
  SinCos/2 -> Product2/2, Product10/1
  smith_norm/1 -> smith normalization/1
  Product4/1 -> Product3/2, Product11/2
  smith normalization/1 -> Product7/2, Product4/2
  "correct_h "/1 -> h_factor _correc/1
  n (loops)/1 -> h_factor _correc/2, smith normalization/2, dP_nm/2, P_nm/2, g_factor _correct/2, h_n^m1/2, g_n^m/2
  Sum3/1 -> g_n^m/3, h_factor _correc/3, g_factor _correct/3, smith normalization/3, dP_nm/3, P_nm/3, h_n^m1/3
  correct_g/1 -> g_factor _correct/1
  Constant1/1 -> Divide/2
  days/1 -> Divide/1
  g_factor _correct/1 -> Product6/1
  Divide/1 -> Product5/2, Product6/2
  h_factor _correc/1 -> Product5/1
  Sum5/1 -> Product1/1, Product10/2
  h_n^m1/1 -> Sum5/1
  Product5/1 -> Sum5/2
  Sum6/1 -> Product2/1, Product9/2
  g_n^m/1 -> Sum6/1
  Product6/1 -> Sum6/2
  dP_nm/1 -> Product7/1
  Product7/1 -> Product8/2
  Product8/1 -> Sum1/1
  SinCos/1 -> Product9/1, Product1/2
  Product10/1 -> Sum7/2
  Product9/1 -> Sum7/1
  Sum7/1 -> Product11/1
  Product11/1 -> Product12/1
  Product12/1 -> Sum2/1

== system verificationGG/ENVIRONMENT/Magnetic Torque/MAGNETIC TORQUE in BODY/B in ECI system/spherical coordinates/Subsystem/If Action Subsystem ==
  In1 : Inport
  Action Port : ActionPort  ActionPortLabel=if(u1 ==0)
  Constant : Constant  Value=0.0000001
  Sum : Sum  Inputs=|++
  Out1 : Outport
  wires:
  In1/1 -> Sum/1
  Sum/1 -> Out1/1
  Constant/1 -> Sum/2

== system verificationGG/ENVIRONMENT/Magnetic Torque/MAGNETIC TORQUE in BODY/B in ECI system/spherical coordinates/Subsystem/If Action Subsystem1 ==
  In1 : Inport
  Action Port : ActionPort  ActionPortLabel=elseif(u1==pi)
  Constant : Constant  Value=0.0000001
  Sum : Sum  Inputs=|++
  Out1 : Outport
  wires:
  In1/1 -> Sum/1
  Sum/1 -> Out1/1
  Constant/1 -> Sum/2

== system verificationGG/ENVIRONMENT/Magnetic Torque/MAGNETIC TORQUE in BODY/B in ECI system/spherical coordinates/Subsystem/If Action Subsystem2 ==
  In1 : Inport
  Action Port : ActionPort  ActionPortLabel=else
  Out1 : Outport
  wires:
  In1/1 -> Out1/1

== matlab function verificationGG/ENVIRONMENT/Magnetic Torque/MAGNETIC TORQUE in BODY/B in ECI system/spherical coordinates/Subsystem/P(v) ==
  data: u input; y output
function y = fcn(u)

P=@(v) [ cos(v)                         sin(v)                               0                             0                   0 
        (3*cos(v)^2-1)/2                3*cos(v)*sin(v)                      3*sin(v)^2                    0                   0
        (5*cos(v)^3-3*cos(v))/2         sin(v)*(15*cos(v)^2-3)/2             15*cos(v)*sin(v)^2            sin(v)^3*15         0
        (35*cos(v)^4-30*cos(v)^2+3)/8   sin(v)*(140*cos(v)^3-60*cos(v))/8    sin(v)^2*(420*cos(v)^2-60)/8  105*sin(v)^3*cos(v) 105*sin(v)^4  ];


y = P(u);

== matlab function verificationGG/ENVIRONMENT/Magnetic Torque/MAGNETIC TORQUE in BODY/B in ECI system/spherical coordinates/Subsystem/dP(v) ==
  data: u input; y output
function y = fcn(u)

dP=@(v) [-sin(v)                                cos(v)                                                          0                                                          0                                  0
         -3*sin(v)*cos(v)                       3*(cos(v)^2-sin(v)^2)                                           6*sin(v)*cos(v)                                            0                                  0
         (-15*cos(v)^2+3)/2*sin(v)              (15*cos(v)^2-3)/2*cos(v)-sin(v)^2*(15*cos(v))                   30*cos(v)^2*sin(v)-15*sin(v)^3                             45*cos(v)*sin(v)^2                 0
         -sin(v)*(140*cos(v)^3-60*cos(v))/8     cos(v)*(140*cos(v)^3-60*cos(v))/8-sin(v)^2*(420*cos(v)^2-60)/8  2*sin(v)*cos(v)*(420*cos(v)^2-60)/8-sin(v)^3*(105*cos(v))  105*(3*sin(v)^2*cos(v)^2-sin(v)^4) 420*sin(v)^3*cos(v)];

y = dP(u);
